simulink model "Controler"  (R2021a)
settings: Solver=VariableStepAuto  StartTime=0.0  StopTime=10.0  RelTol=1e-3
settings Model: DataDictionary=Thermostat.sldd  Creator=smrh1  LastModifiedBy=smrh1

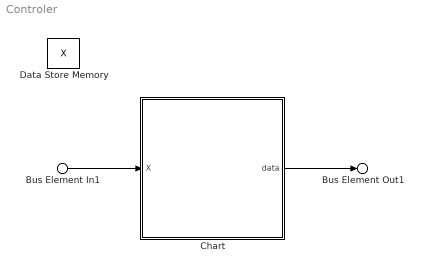
== system Controler ==
  Bus Element In1 : Inport  PortName=X
  Chart : Stateflow chart  TreatAsAtomicUnit=on
  Data Store Memory : DataStoreMemory  DataStoreName=X  ReadBeforeWriteMsg=warning  WriteAfterWriteMsg=warning  WriteAfterReadMsg=warning  InitialValue=[16.5,16.5,16.5,16.5]  ShowAdditionalParam=off
  Bus Element Out1 : Outport  PortName=H
  wires:
  Bus Element In1/1 -> Chart/1(X)
  Chart/1(data) -> Bus Element Out1/1

== stateflow chart Controler/Chart ==
  state st13
    entry:
    h2 = 0;
    h4 = 0;
    Room=[1,3];
    state s1 [parallel]
      settings: executionOrder=1
      state s1_on
        entry:
        h1 = 1
      state s1_off
        entry:
        h1 = 0
      (default) -> st13.s1.s1_on
      st13.s1.s1_on -> st13.s1.s1_off : [x(1)>=off(1)]
      st13.s1.s1_off -> st13.s1.s1_on : [x(1)<=on(1)]
    state s3 [parallel]
      settings: executionOrder=2
      state s3_on
        entry:
        h3 = 1
      state s3_off
        entry:
        h3 = 0
      (default) -> st13.s3.s3_on
      st13.s3.s3_on -> st13.s3.s3_off : [x(3)>=off(3)]
      st13.s3.s3_off -> st13.s3.s3_on : [x(3)<=on(3)]
  state st14
    entry:
    h2 = 0;
    h3 = 0;
    Room=[1,4];
    state s1 [parallel]
      settings: executionOrder=1
      state s1_on
        entry:
        h1 = 1
      state s1_off
        entry:
        h1 = 0
      (default) -> st14.s1.s1_on
      st14.s1.s1_on -> st14.s1.s1_off : [x(1)>=off(1)]
      st14.s1.s1_off -> st14.s1.s1_on : [x(1)<=on(1)]
    state s4 [parallel]
      settings: executionOrder=2
      state s4_on
        entry:
        h4 = 1
      state s4_off
        entry:
        h4 = 0
      (default) -> st14.s4.s4_on
      st14.s4.s4_on -> st14.s4.s4_off : [x(4)>=off(4)]
      st14.s4.s4_off -> st14.s4.s4_on : [x(4)<=on(4)]
  state st12
    entry:
    h3 = 0;
    h4 = 0;
    Room=[1,2];
    state s1 [parallel]
      settings: executionOrder=1
      state s1_on1
        entry:
        h1 = 1
      state s1_off
        entry:
        h1 = 0
      (default) -> s1_on1
      s1_on1 -> st12.s1.s1_off : [x(1)>=off(1) ]
      st12.s1.s1_off -> s1_on1 : [x(1)<=on(1) ]
    state s2 [parallel]
      settings: executionOrder=2
      state s2_on
        entry:
        h2 = 1
      state s1_off1
        entry:
        h2 = 0
      (default) -> st12.s2.s2_on
      st12.s2.s2_on -> s1_off1 : [x(2)>=off(2)]
      s1_off1 -> st12.s2.s2_on : [x(2)<=on(2)]
  state st24
    entry:
    h1 = 0;
    h3 = 0;
    Room=[1,3];
    state s2 [parallel]
      settings: executionOrder=1
      state s2_on
        entry:
        h2 = 1
      state s2_off
        entry:
        h2 = 0
      (default) -> st24.s2.s2_on
      st24.s2.s2_on -> s2_off : [x(2)>=off(2)]
      s2_off -> st24.s2.s2_on : [x(2)<=on(2)]
    state s4 [parallel]
      settings: executionOrder=2
      state s4_on
        entry:
        h4 = 1
      state s4_off
        entry:
        h4 = 0
      (default) -> st24.s4.s4_on
      st24.s4.s4_on -> st24.s4.s4_off : [x(4)>=off(4)]
      st24.s4.s4_off -> st24.s4.s4_on : [x(4)<=on(4)]
  state st34
    entry:
    h1 = 0;
    h2 = 0;
    Room=[3,4];
    state s3 [parallel]
      settings: executionOrder=1
      state s3_on
        entry:
        h3 = 1
      state s3_off
        entry:
        h3 = 0
      (default) -> st34.s3.s3_on
      st34.s3.s3_on -> st34.s3.s3_off : [x(3)>=off(3)]
      st34.s3.s3_off -> st34.s3.s3_on : [x(3)<=on(3)]
    state s4 [parallel]
      settings: executionOrder=2
      state s4_on
        entry:
        h4 = 1
      state s4_off
        entry:
        h4 = 0
      (default) -> st34.s4.s4_on
      st34.s4.s4_on -> st34.s4.s4_off : [x(4)>=off(4)]
      st34.s4.s4_off -> st34.s4.s4_on : [x(4)<=on(4)]
  state st23
    entry:
    h1 = 0;
    h4 = 0;
    Room=[2,3];
    state s2 [parallel]
      settings: executionOrder=1
      state s2_on
        entry:
        h2 = 1;
      state s1_off
        entry:
        h2 = 0;
      (default) -> st23.s2.s2_on
      st23.s2.s2_on -> st23.s2.s1_off : [x(2)>= off(2)]
      st23.s2.s1_off -> st23.s2.s2_on : [x(2)<=on(2)]
    state s3 [parallel]
      settings: executionOrder=2
      state s3_on
        entry:
        h3 = 1;
      state s3_off
        entry:
        h3 = 0;
      (default) -> st23.s3.s3_on
      st23.s3.s3_on -> st23.s3.s3_off : [x(3)>=off(3)]
      st23.s3.s3_off -> st23.s3.s3_on : [x(3)<=on(3) ]
  state start
    entry:
    h1=0
    h4=0
    h2=1;
    h3=1;
  st13 -> st14 [order 2] : [x(3)-x(4)>=dif(4) & x(4)<=get(4)]{h1=0;h3=0}
  st12 -> st13 [order 1] : [x(2)-x(3)>=dif(3) & x(3)<=get(3)]{h1=0;h2=0;}
  st13 -> st12 [order 1] : [x(3)-x(2)>=dif(2) & x(2)<=get(2)]{h1=0;h3=0;}
  st14 -> st13 [order 1] : [x(4)-x(3)>=dif(3) & x(3)<=get(3)]{h1=0;h4=0;}
  st13 -> st23 [order 3] : [(x(1)-x(2)>=dif(2) & x(2)<=get(2))]{h1=0;h3=0;}
  st13 -> st34 [order 4] : [x(1)-x(4)>=dif(4) & x(4)<=get(4)]{h1=0;h3=0;}
  st23 -> st13 [order 2] : [(x(2)-x(1)>=dif(1) & x(1)<=get(1))]{h2=0;h3=0}
  st34 -> st13 [order 1] : [x(4)-x(1)>=dif(1) & x(1)<=get(1)]{h3=0;h4=0;}
  st12 -> st14 [order 3] : [x(2)-x(4)>=dif(4) & x(4)<=get(4)]{h1=0;h2=0;}
  st14 -> st12 [order 2] : [x(4)-x(2)>=dif(2) & x(2)<=get(2)]{h1=0;h4=0;}
  st14 -> st34 [order 4] : [x(1)-x(3)>=dif(3) & x(3)<=get(3)]{h1=0;h4=0;}
  st14 -> st24 [order 3] : [x(4)-x(2)>=dif(2) & x(2)<=get(2)]{h1=0;h4=0;}
  st24 -> st14 [order 2] : [x(2)-x(4)>=dif(4) & x(4)<=get(4)]{h2=0;h4=0;}
  st34 -> st14 [order 2] : [x(3)-x(1)>=dif(1) & x(1)<=get(1)]{h3=0;h4=0;}
  st12 -> st23 [order 2] : [x(1)-x(3)>=dif(3) & x(3)<=get(3)]{h1=0;h2=0;}
  st23 -> st12 [order 1] : [x(3)-x(1)>=dif(1) & x(1)<=get(1)]{h2=0;h3=0;}
  st24 -> st12 [order 1] : [x(4)-x(1)>=dif(1) & x(1)<=get(1)]{h2=0;h4=0;}
  st12 -> st24 [order 4] : [x(1)-x(4)>=dif(4) & x(4)<=get(4)]{h1=0;h2=0;}
  (default) -> start
  start -> st23
  st23 -> st24 [order 3] : [x(3)-x(4)>=dif(4) & x(4)<=get(4)]{h2=0;h3=0;}
  st24 -> st34 [order 4] : [x(2)-x(3)>=dif(3) & x(3)<=get(3)]{h2=0;h4=0;}
  st24 -> st23 [order 3] : [x(4)-x(3)>=dif(3) & x(3)<=get(3)]{h2=0;h4=0;}
  st34 -> st24 [order 4] : [x(3)-x(2)>=dif(2) & x(2)<=get(2)]{h3=0;h4=0;}
  st23 -> st34 [order 4] : [x(2)-x(4)>=dif(4) & x(4)<=get(4)]{h3=0;h2=0;}
  st34 -> st23 [order 3] : [x(4)-x(2)>=dif(2) & x(2)<=get(2)]{h3=0;h4=0;}
  data: X input; data output
